simulink model "just_observer"  (R2022b)
settings: Solver=VariableStepAuto  StartTime=0.0  StopTime=10.0  RelTol=1e-3
values from neighbouring files (symbols this model uses):
  L = acker(A', C', [so so so])    [params.m]
undefined symbols (not defined in the file or in its folder): A, C
settings Model: Creator=antekgrajek  LastModifiedBy=antekgrajek

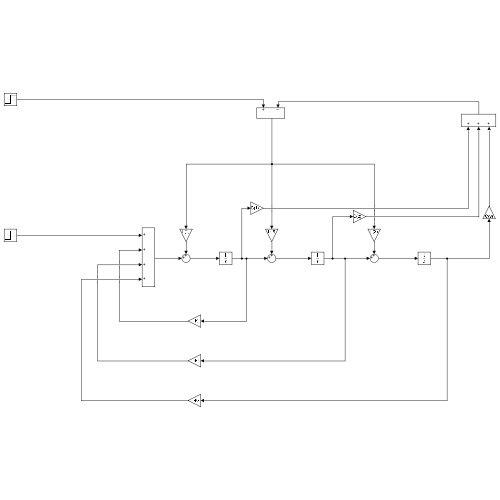
[thumbnail: Simulink's stored preview of the top-level diagram]
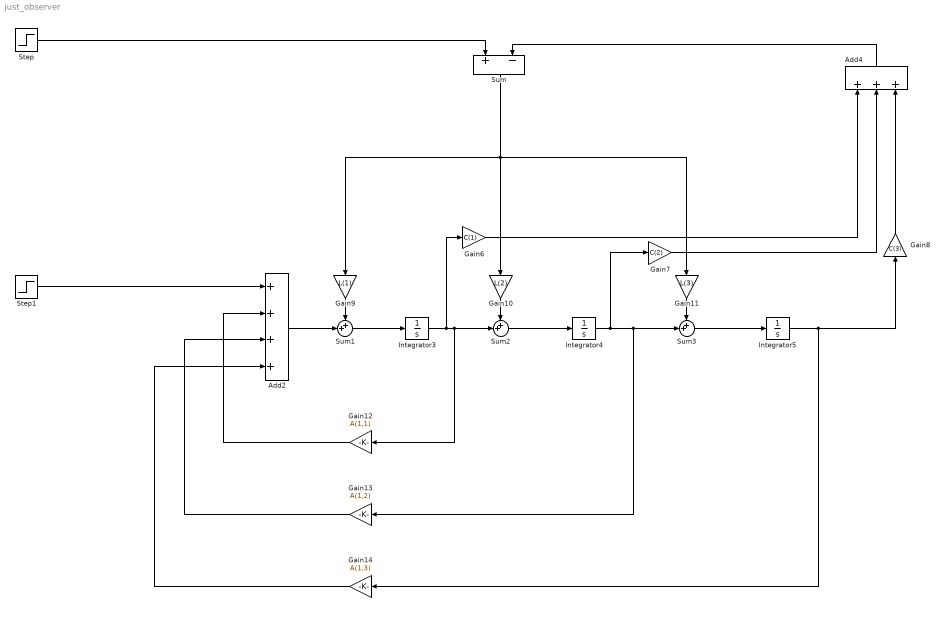
== system just_observer ==
  Add2 : Sum  Inputs=++++
  Add4 : Sum  Inputs=+++
  Gain10 : Gain  Gain=L(2)
  Gain11 : Gain  Gain=L(3)
  Gain12 : Gain  Gain=A(1,1)
  Gain13 : Gain  Gain=A(1,2)
  Gain14 : Gain  Gain=A(1,3)
  Gain6 : Gain  Gain=C(1)
  Gain7 : Gain  Gain=C(2)
  Gain8 : Gain  Gain=C(3)
  Gain9 : Gain  Gain=L(1)
  Integrator3 : Integrator  InitialCondition=10
  Integrator4 : Integrator  InitialCondition=20
  Integrator5 : Integrator  InitialCondition=30
  Step : Step  SampleTime=0
  Step1 : Step  SampleTime=0
  Sum : Sum  Inputs=+-
  Sum1 : Sum  Inputs=++|
  Sum2 : Sum  Inputs=++|
  Sum3 : Sum  Inputs=++|
  wires:
  Integrator3/1 -> Gain6/1, Gain12/1, Sum2/2
  Sum3/1 -> Integrator5/1
  Integrator5/1 -> Gain14/1, Gain8/1
  Gain7/1 -> Add4/2
  Add2/1 -> Sum1/2
  Sum2/1 -> Integrator4/1
  Gain14/1 -> Add2/4
  Gain11/1 -> Sum3/1
  Gain6/1 -> Add4/1
  Sum1/1 -> Integrator3/1
  Add4/1 -> Sum/2
  Gain13/1 -> Add2/3
  Sum/1 -> Gain11/1, Gain10/1, Gain9/1
  Integrator4/1 -> Gain7/1, Gain13/1, Sum3/2
  Gain10/1 -> Sum2/1
  Gain8/1 -> Add4/3
  Gain9/1 -> Sum1/1
  Gain12/1 -> Add2/2
  Step1/1 -> Add2/1
  Step/1 -> Sum/1
